simulink model "REALTIME_PART1_discretefeedforward"  (R2020b)
settings: Solver=ode3  StartTime=0.0  StopTime=5  FixedStep=0.001  RelTol=1e-3
values from neighbouring files (symbols this model uses):
  denHwa = [1 177.715317526 15791.3670417]    [filters.mat]
  denHws = [1 177.715317526 15791.3670417]    [filters.mat]
  numHwa = [0 15791.3670417 0]    [filters.mat]
  numHws = [0 15791.3670417 0]    [filters.mat]
undefined symbols (not defined in the file or in its folder): BEMF_comp, Beq_hat, ctrl, degs2rpm, DiscIntNeverNeededParam, friction_comp, gbox, inertia_comp, K_w, National_Instruments, PCI, rpm2rads, sens, T, tau_hat, Tl
libraries: sldrtlib x2, simulink x1
settings Model: ExtModeTrigDuration=6000  Creator=gioel  LastModifiedBy=pavarinlau
settings DataIOCC: ReturnWorkspaceOutputs=off
settings RTWCC: Description=Simulink Desktop Real-Time  SystemTargetFile=sldrt.tlc  TemplateMakefile=sldrt.tmf  RTWCompilerOptimization=on
settings CodeAppCC: MaxIdLength=95
settings SimulinkDesktopRealTimeCC: TargetPreCompLibLocation=C:\Program Files\MATLAB\R2020b\toolbox\sldrt\lib\win64

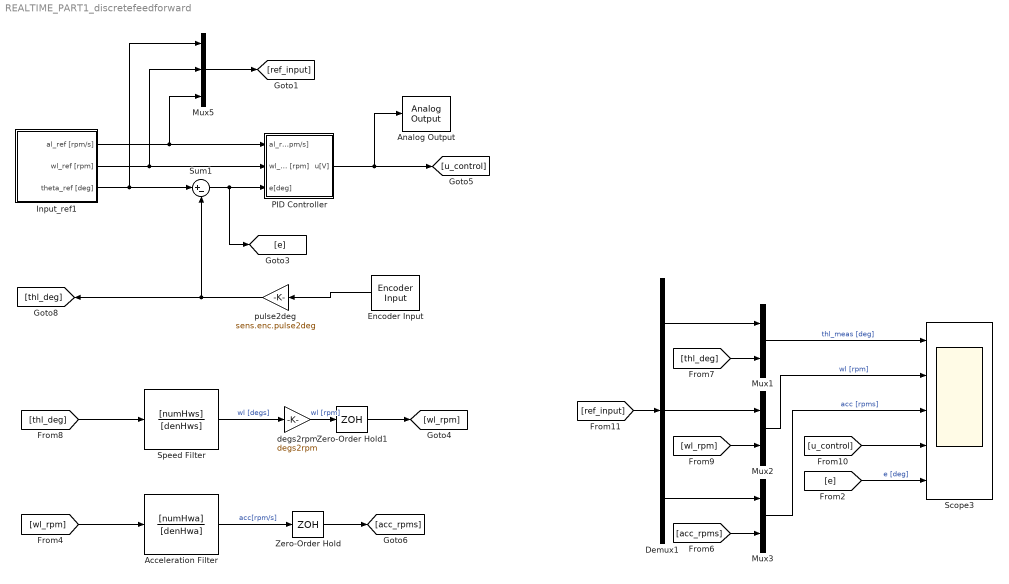
== system REALTIME_PART1_discretefeedforward ==
  Acceleration Filter : TransferFcn  Numerator=[numHwa]  Denominator=[denHwa]
  Analog Output : sldrtlib/Analog Output  SampleTime=-1  MaxMissedTicks=10  ShowMissedTicks=off  YieldWhenWaiting=off  DrvName=National_Instruments/PCI-6221  DrvAddress=4294967295  DrvOptions=[0 0 0 2 0]  Channels=1  RangeMode=1  VoltRange=1  InitialValue=0  FinalValue=0
      settings: AttributesFormatString=National Instruments\nPCI-6221 [auto]
  Demux1 : Demux  Outputs=3
  Encoder Input : sldrtlib/Encoder Input  SampleTime=T  MaxMissedTicks=10  ShowMissedTicks=off  YieldWhenWaiting=off  DrvName=National_Instruments/PCI-6221  DrvAddress=4294967295  DrvOptions=[0 0 0 2 0]  Channels=1  QuadMode=3  IndexPulse=2  InputFilter=Inf  DataType=1
      settings: AttributesFormatString=National Instruments\nPCI-6221 [auto]
  Input_ref1 : Subsystem
  Mux1 : Mux  Inputs=2
  Mux2 : Mux  Inputs=2
  Mux3 : Mux  Inputs=2
  Mux5 : Mux  Inputs=3
  PID Controller : Subsystem
  Scope3 : Scope  NumInputPorts=5
  Speed Filter : TransferFcn  Numerator=[numHws]  Denominator=[denHws]
  Sum1 : Sum  Inputs=|+-
  Zero-Order Hold : ZeroOrderHold  SampleTime=T
  Zero-Order Hold1 : ZeroOrderHold  SampleTime=T
  degs2rpm : Gain  Gain=degs2rpm
  pulse2deg : Gain  Gain=sens.enc.pulse2deg
  wires:
  Sum1/1 -> [e], PID Controller/3(e[deg])
  PID Controller/1(u[V]) -> Analog Output/1, [u_control]
  pulse2deg/1 -> [thl_deg], Sum1/2
  Demux1/1 -> Mux1/1
  Mux2/1 -> Scope3/2  "wl [rpm]"
  Demux1/2 -> Mux2/1
  [ref_input] -> Demux1/1
  [wl_rpm] -> Acceleration Filter/1
  [wl_rpm] -> Mux2/2
  Mux3/1 -> Scope3/3  "acc [rpms]"
  [thl_deg] -> Speed Filter/1
  [u_control] -> Scope3/4
  Acceleration Filter/1 -> Zero-Order Hold/1  "acc[rpm/s]"
  Speed Filter/1 -> degs2rpm/1  "wl [degs]"
  [acc_rpms] -> Mux3/2
  degs2rpm/1 -> Zero-Order Hold1/1  "wl [rpm]"
  Mux1/1 -> Scope3/1  "thl_meas [deg]"
  [thl_deg] -> Mux1/2
  Demux1/3 -> Mux3/1
  [e] -> Scope3/5  "e [deg]"
  Input_ref1/1(al_ref [rpm/s]) -> Mux5/3, PID Controller/1("al_ref [rpm/s]  ")
  Input_ref1/3(theta_ref [deg]) -> Mux5/1, Sum1/1
  Mux5/1 -> [ref_input]
  Input_ref1/2(wl_ref [rpm]) -> Mux5/2, PID Controller/2("wl_ref [rpm] ")
  Encoder Input/1 -> pulse2deg/1
  Zero-Order Hold/1 -> [acc_rpms]
  Zero-Order Hold1/1 -> [wl_rpm]

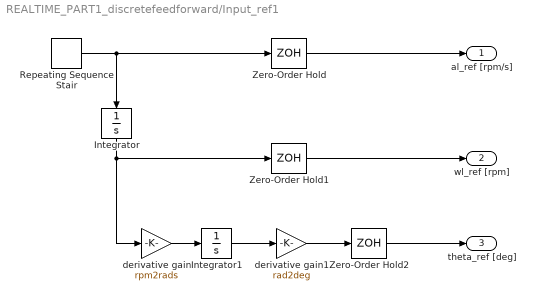
== system REALTIME_PART1_discretefeedforward/Input_ref1 ==
  Integrator : Integrator
  Integrator1 : Integrator
  Repeating Sequence Stair : simulink/Sources/Repeating Sequence Stair  OutValues=[900 0 -900 -900 0 900].'  tsamp=0.5  OutMin=[]  OutMax=[]  OutDataTypeStr=double  OutputDataTypeScalingMode=double  OutDataType=fixdt(0,8)  ConRadixGroup=Best Precision: Vector-wise  OutScaling=2^-12
  Zero-Order Hold : ZeroOrderHold  SampleTime=T
  Zero-Order Hold1 : ZeroOrderHold  SampleTime=T
  Zero-Order Hold2 : ZeroOrderHold  SampleTime=T
  derivative gain : Gain  Gain=rpm2rads
  derivative gain1 : Gain  Gain=rad2deg
  al_ref [rpm/s] : Outport  VectorParamsAs1DForOutWhenUnconnected=off
  wl_ref [rpm] : Outport  Port=2  VectorParamsAs1DForOutWhenUnconnected=off
  theta_ref [deg] : Outport  Port=3  VectorParamsAs1DForOutWhenUnconnected=off
  wires:
  Integrator/1 -> derivative gain/1, Zero-Order Hold1/1
  derivative gain/1 -> Integrator1/1
  derivative gain1/1 -> Zero-Order Hold2/1
  Integrator1/1 -> derivative gain1/1
  Repeating Sequence Stair/1 -> Integrator/1, Zero-Order Hold/1
  Zero-Order Hold/1 -> al_ref [rpm/s]/1
  Zero-Order Hold1/1 -> wl_ref [rpm]/1
  Zero-Order Hold2/1 -> theta_ref [deg]/1

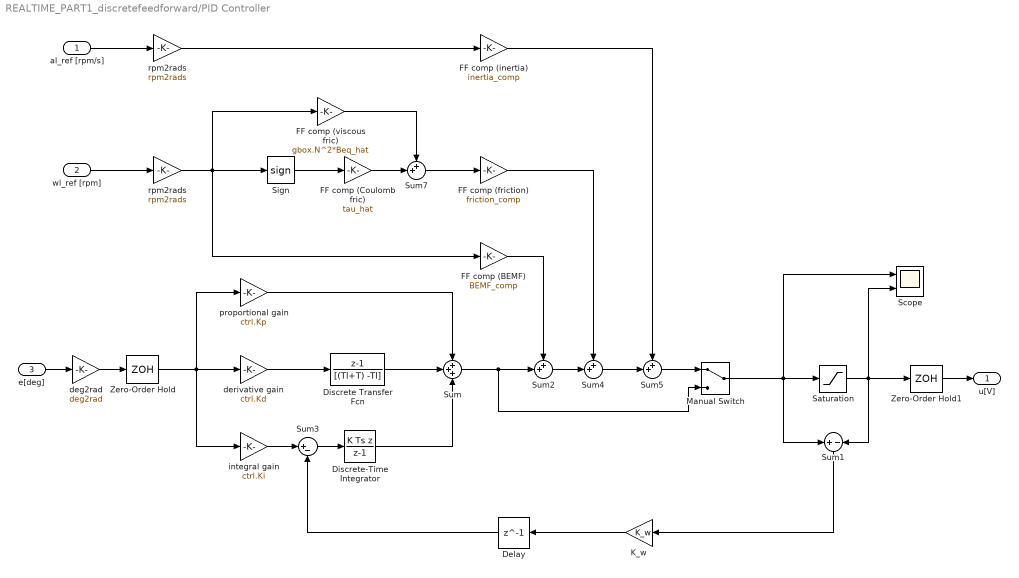
== system REALTIME_PART1_discretefeedforward/PID Controller ==
  "al_ref [rpm/s]  " : Inport
  "wl_ref [rpm] " : Inport  Port=2
  e[deg] : Inport  Port=3
  Delay : Delay  DelayLength=1  InitialCondition=0
  Discrete Transfer Fcn : DiscreteTransferFcn  Numerator=[1 -1]  Denominator=[(Tl+T) -Tl]
  Discrete-Time Integrator : DiscreteIntegrator  IntegratorMethod=Integration: Backward Euler  SampleTime=T  ICPrevOutput=DiscIntNeverNeededParam  ICPrevScaledInput=DiscIntNeverNeededParam
  FF comp (Coulomb fric) : Gain  Gain=tau_hat
  FF comp (viscous fric) : Gain  Gain=gbox.N^2*Beq_hat
  FF comp (BEMF) : Gain  Gain=BEMF_comp
  FF comp (friction) : Gain  Gain=friction_comp
  FF comp (inertia) : Gain  Gain=inertia_comp
  "K_w " : Gain  Gain=K_w
  Manual Switch : ManualSwitch
  Saturation : Saturate  UpperLimit=10  LowerLimit=-10
  Scope : Scope  NumInputPorts=2
  "Sign " : Signum  ZeroCross=off
  Sum : Sum  Inputs=+++
  Sum1 : Sum  Inputs=+|-
  Sum{2,4..5,7} (4 alike) : Sum  Inputs=++|
  Sum3 : Sum  Inputs=|+-
  Zero-Order Hold : ZeroOrderHold  SampleTime=T
  Zero-Order Hold1 : ZeroOrderHold  SampleTime=T
  deg2rad : Gain  Gain=deg2rad
  derivative gain : Gain  Gain=ctrl.Kd
  integral gain : Gain  Gain=ctrl.Ki
  proportional gain : Gain  Gain=ctrl.Kp
  rpm2rads : Gain  Gain=rpm2rads
  "rpm2rads " : Gain  Gain=rpm2rads
  u[V] : Outport
  wires:
  proportional gain/1 -> Sum/1
  Saturation/1 -> Scope/2, Zero-Order Hold1/1, Sum1/2
  Zero-Order Hold1/1 -> u[V]/1
  e[deg]/1 -> deg2rad/1
  deg2rad/1 -> Zero-Order Hold/1
  Zero-Order Hold/1 -> integral gain/1, derivative gain/1, proportional gain/1
  derivative gain/1 -> Discrete Transfer Fcn/1
  Discrete Transfer Fcn/1 -> Sum/2
  Discrete-Time Integrator/1 -> Sum/3
  Sum1/1 -> "K_w "/1
  integral gain/1 -> Sum3/1
  Sum3/1 -> Discrete-Time Integrator/1
  "K_w "/1 -> Delay/1
  Manual Switch/1 -> Sum1/1, Scope/1, Saturation/1
  Sum2/1 -> Sum4/2
  Sum/1 -> Manual Switch/2, Sum2/2
  Sum4/1 -> Sum5/2
  Sum5/1 -> Manual Switch/1
  "al_ref [rpm/s]  "/1 -> rpm2rads/1
  Sum7/1 -> FF comp (friction)/1
  FF comp (viscous fric)/1 -> Sum7/1
  "wl_ref [rpm] "/1 -> "rpm2rads "/1
  FF comp (inertia)/1 -> Sum5/1
  "rpm2rads "/1 -> "Sign "/1, FF comp (viscous fric)/1, FF comp (BEMF)/1
  FF comp (Coulomb fric)/1 -> Sum7/2
  rpm2rads/1 -> FF comp (inertia)/1
  "Sign "/1 -> FF comp (Coulomb fric)/1
  FF comp (friction)/1 -> Sum4/1
  FF comp (BEMF)/1 -> Sum2/1
  Delay/1 -> Sum3/2
